simulink model "lab3"  (R2019b)
settings: Solver=VariableStepAuto  StartTime=0.0  StopTime=time  RelTol=1e-3
values from neighbouring files (symbols this model uses):
  deltat = 0.01    [main.m]
  Dumax = 20    [main.m]
  Dumin = -20    [main.m]
  Gs = tf([b1 b0], [1 a1 a0])    [main.m]
  Kc = 0.0065    [PI_contrller.m]    (also in main.m = pid.Kc)
  pid = PID(I0, c2, c1, c0)    [main.m]
  tauD = pid.tauD    [main.m]
  tauf = pid.tauF    [main.m]
  tauI = 244.5    [PI_contrller.m]    (also in main.m = pid.tauI)
  Umax = 5    [main.m]
  Umin = -7    [main.m]
libraries: simulink x3
settings Model: Creator=adityaaaap  LastModifiedBy=adityaaaap

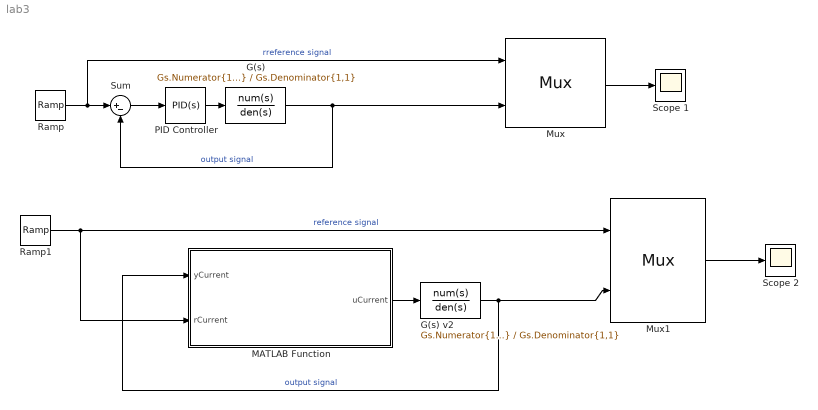
== system lab3 ==
  G(s) : TransferFcn  Numerator=Gs.Numerator{1,1}  Denominator=Gs.Denominator{1,1}
  "G(s) v2 " : TransferFcn  Numerator=Gs.Numerator{1,1}  Denominator=Gs.Denominator{1,1}
  MATLAB Function : MATLAB Function  TreatAsAtomicUnit=on
  Mux : Mux  Inputs=2
      settings: DisplayOption=signals
  Mux1 : Mux  Inputs=2
      settings: DisplayOption=signals
  PID Controller : simulink/Continuous/PID Controller  Controller=PID  Form=Parallel  TimeDomain=Continuous-time  SampleTime=-1  IntegratorMethod=Forward Euler  FilterMethod=Forward Euler  ControllerParametersSource=internal  P=pid.P  I=pid.I  D=pid.D  UseFilter=on  N=pid.N  TunerSelectOption=Transfer Function Based (PID Tuner App)  InitialConditionSource=internal  InitialConditionForIntegrator=0  InitialConditionForFilter=0  DifferentiatorICPrevScaledInput=0  ExternalReset=none  TrackingMode=off  Kt=1  LimitOutput=off  UpperSaturationLimit=inf  LowerSaturationLimit=-inf  LinearizeAsGain=on  AntiWindupMode=none  Kb=1  POutMin=[]  POutMax=[]  IOutMin=[]  IOutMax=[]  DOutMin=[]  DOutMax=[]  NOutMin=[]  NOutMax=[]  SumOutMin=[]  SumOutMax=[]  SaturationOutMin=[]  SaturationOutMax=[]  PParamMin=[]  PParamMax=[]  IParamMin=[]  IParamMax=[]  DParamMin=[]  DParamMax=[]  NParamMin=[]  NParamMax=[]  KbParamMin=[]  KbParamMax=[]  KtParamMin=[]  KtParamMax=[]  KbOutMin=[]  KbOutMax=[]  KtOutMin=[]  KtOutMax=[]  IntegratorOutMin=[]  IntegratorOutMax=[]  FilterOutMin=[]  FilterOutMax=[]  SumI1OutMin=[]  SumI1OutMax=[]  SumI2OutMin=[]  SumI2OutMax=[]  SumI3OutMin=[]  SumI3OutMax=[]  SumI4OutMin=[]  SumI4OutMax=[]  SumDOutMin=[]  SumDOutMax=[]  DifferentiatorOutMin=[]  DifferentiatorOutMax=[]  FilterDiffOutCoefMin=[]  FilterDiffOutCoefMax=[]  ReciprocalOutMin=[]  ReciprocalOutMax=[]  SumDenOutMin=[]  SumDenOutMax=[]  SumNumOutMin=[]  SumNumOutMax=[]  DivideOutMin=[]  DivideOutMax=[]  IntegratorContinuousStateAttributes=''  IntegratorStateMustResolveToSignalObject=off  IntegratorRTWStateStorageClass=Auto  FilterContinuousStateAttributes=''  FilterStateMustResolveToSignalObject=off  FilterRTWStateStorageClass=Auto  ParallelPVariant=InternalParameters  IdealPVariant=Disabled  IVariant=InternalParameters  DVariant=InternalParameters  IntegratorVariant=Continuous  SatVariant=Disabled  AWVariant=Passthrough  PCopyVariant=Disabled  TRVariant=Disabled  FdbkBlocksVariant=Forward  IdealPFdbkVariant=Disabled  SatFdbkVariant=Disabled  DerivativeFilterVariant=ContFilter  NVariant=InternalParameters  NCopyVariant=Disabled  FilterICVariant=InternalICsFilter  IntegratorICVariant=InternalICs  ExternalResetVariant=Disabled  TRSumVariant=Passthrough  SumFdbkVariant=Disabled  SumVariant=Sum_PID
  Ramp : simulink/Sources/Ramp  slope=1  start=0  InitialOutput=0
  Ramp1 : simulink/Sources/Ramp  slope=1  start=0  InitialOutput=0
  "Scope 1 " : Scope
  "Scope 2 " : Scope
  Sum : Sum  Inputs=|+-
  wires:
  Ramp/1 -> Mux/1, Sum/1  "rreference signal"
  Sum/1 -> PID Controller/1
  PID Controller/1 -> G(s)/1
  G(s)/1 -> Mux/2, Sum/2  "output signal"
  Mux/1 -> "Scope 1 "/1
  MATLAB Function/1(uCurrent) -> "G(s) v2 "/1
  "G(s) v2 "/1 -> MATLAB Function/1(yCurrent), Mux1/2  "output signal"
  Mux1/1 -> "Scope 2 "/1
  Ramp1/1 -> Mux1/1, MATLAB Function/2(rCurrent)  "reference signal"

== matlab function lab3/MATLAB Function ==
  settings: updateMethod=DISCRETE  sampleTime=deltat
  data: yCurrent input; uCurrent output; rCurrent input; Kc parameter; tauI parameter; tauD parameter; tauf parameter; deltat parameter; Umin parameter; Umax parameter; Dumin parameter; Dumax parameter
function uCurrent = PIDV(yCurrent,rCurrent,Kc, tauI, tauD, tauf, deltat, Umin, Umax, Dumin, Dumax)
    persistent uPast 
    if isempty(uPast)
        uPast=0;
    end
    
    persistent yPast 
    if isempty(yPast)
        yPast=0; 
    end
    
    persistent uDPast 
    if isempty(uDPast)
        uDPast=0;
    end
    
    persistent rPast 
    if isempty(rPast)
        rPast=0;
    end
    
    uDCurrent=tauf/(tauf+deltat)*uDPast+(Kc*tauD)/(tauf+deltat)*(yCurrent-yPast);
    
    uCurrent=uPast+Kc*(rCurrent-yCurrent-rPast+yPast)+ (Kc*deltat)/tauI*(rCurrent-yCurrent)-uDCurrent+uDPast;
    
    uCurrent=uPast+Kc*(-yCurrent+yPast)+ (Kc*deltat)/tauI*(rCurrent-yCurrent)-uDCurrent+uDPast;
    Du=(uCurrent-uPast)/deltat;
    
    if (Du>Dumax)
        uCurrent=uPast+Dumax*deltat;
        Du=Dumax;
    end
    
    if (Du<Dumin) 
        uCurrent=uPast+Dumin*deltat;
        Du=Dumin; 
    end
    
    if (uCurrent>Umax) 
        uCurrent=Umax;
    end
    
    if (uCurrent<Umin) 
        uCurrent=Umin; 
    end
    
    uDPast=uDCurrent; 
    uPast=uCurrent; 
    yPast=yCurrent; 
    rPast=rCurrent;
end
